simulink model "cvoo_g19_servomecanismo_atuador"  (R2022a)
settings: Solver=VariableStepAuto  StartTime=0.0  StopTime=100  RelTol=1e-3
values from neighbouring files (symbols this model uses):
  b_h_pt = [ ... (first row only)    [Ponto3.m]    (also in main.m; main_novo.m)
  c_h_pt = eye(size(a_h_pt))    [Ponto3.m]    (also in main.m; main_novo.m)
  conv_max = 5    [main.m]    (also in main_novo.m)
  conv_min = 0    [main.m]    (also in main_novo.m)
  conv_rms = 1.5*conv_res    (= 0.000915639116103)    [main.m]    (also in main_novo.m)
  d_h_pt = zeros(size(b_h_pt))    [Ponto3.m]    (also in main.m; main_novo.m)
  deg = pi/180    (= 0.0174532925199)    [Ponto3.m]    (also in def_model.m; def_model_inicial.m; main.m; main_controlo_altitude.m)
  f_amost = 100    [main.m]    (also in main_novo.m)
  G_sensq = (V_max_sensq-V_min_sensq)/(q_max_sensq-q_min_sensq)    (= 0.006)    [main.m]    (also in main_novo.m)
  Gp_din = (v_pdin_max-v_pdin_min)/(pdin_max-pdin_min)    (= 0.00125)    [main.m]    (also in main_novo.m)
  h_pt_ref = -4    [Ponto3.m]    (also in main.m = -1; main_novo.m = 0)
  K_lqr = lqr(a_h_pt_int, b_h_pt_int, Q, R)    [Ponto3.m]    (also in main.m; main_controlo_altitude.m = lqr(a_h_int, b_h_sf_int, Q, R); main_novo.m)
  offset_pdin = 2.5    [main.m]    (also in main_novo.m)
  Offset_sensq = 2.5    [main.m]    (also in main_novo.m)
  p_din_tau = 0.01    [main.m]    (also in main_novo.m)
  pdin_max = 2e3    (= 2000)    [main.m]    (also in main_novo.m)
  pdin_min = -2e3    (= -2000)    [main.m]    (also in main_novo.m)
  q_max_sensq = 300    [main.m]    (also in main_novo.m)
  q_min_sensq = -300    [main.m]    (also in main_novo.m)
  rad = 180/pi    (= 57.2957795131)    [Ponto3.m]    (also in main.m; main_controlo_altitude.m; main_novo.m)
  rho0 = 1.225    [main.m]    (also in main_novo.m)
  rms_sensq = 4.4    [main.m]    (also in main_novo.m)
  tau = 0.1    [main.m]    (also in main_novo.m)
  u_ref = 1.5    [Ponto3.m]    (also in main.m = 2; main_controlo_altitude.m = -5; main_novo.m = 0)
  vel_max_at = 60    [main.m]    (also in main_novo.m)
  x0 = [0 0 0 0]    [Ponto3.m]    (also in main.m; main_controlo_altitude.m; main_novo.m)
undefined symbols (not defined in the file or in its folder): a_h_pt, cond_ini, max_deflec
libraries: simulink x3
settings Model: Creator=josem  LastModifiedBy=franc
settings SolverCC: AlgebraicLoopSolver=TrustRegion
settings DebuggingCC: UnconnectedInputMsg=warning  UnconnectedOutputMsg=warning  UnconnectedLineMsg=warning  SFMachineParentedDataDiag=warning
settings RTWCC: DLArmComputeVersion=19.05

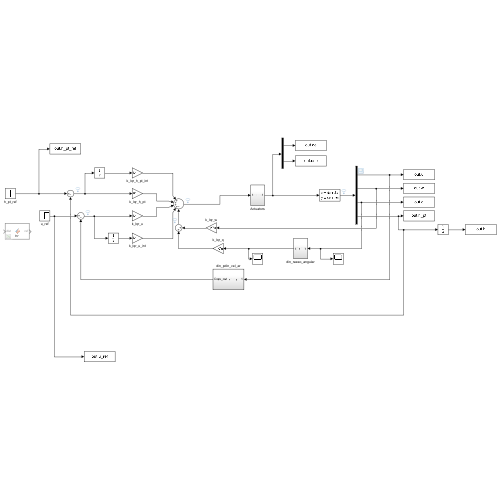
[thumbnail: Simulink's stored preview of the top-level diagram]
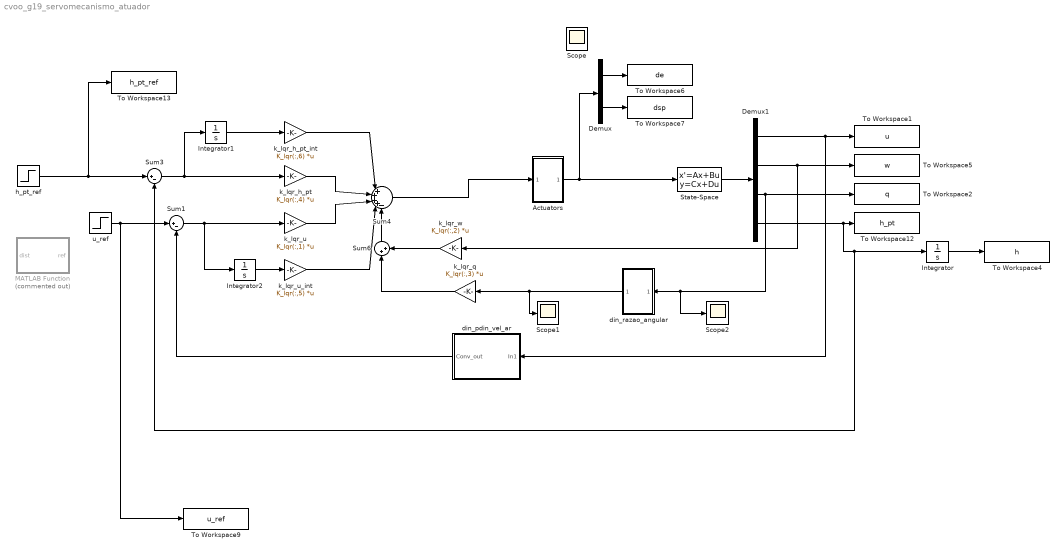
== system cvoo_g19_servomecanismo_atuador ==
  Actuators : Subsystem
  Demux : Demux  Outputs=2
  Demux1 : Demux
  Integrator : Integrator
  Integrator1 : Integrator
  Integrator2 : Integrator
  MATLAB Function : MATLAB Function  Commented=on  TreatAsAtomicUnit=on
  Scope1 : Scope
  Scope2 : Scope
  State-Space : StateSpace  A=a_h_pt  B=b_h_pt  C=c_h_pt  D=d_h_pt  InitialCondition=x0
  Sum1 : Sum  Inputs=|+-
  Sum3 : Sum  Inputs=|+-
  Sum4 : Sum  Inputs=|++++-
  Sum6 : Sum  Inputs=|++
  To Workspace1 : ToWorkspace  VariableName=u  SampleTime=-1
  To Workspace12 : ToWorkspace  VariableName=h_pt  SampleTime=-1
  To Workspace13 : ToWorkspace  VariableName=h_pt_ref  SampleTime=-1
  To Workspace2 : ToWorkspace  VariableName=q  SampleTime=-1
  To Workspace4 : ToWorkspace  VariableName=h  SampleTime=-1
  To Workspace5 : ToWorkspace  VariableName=w  SampleTime=-1
  To Workspace6 : ToWorkspace  VariableName=de  SaveFormat=Structure With Time  SampleTime=-1
  To Workspace7 : ToWorkspace  VariableName=dsp  SaveFormat=Structure With Time  SampleTime=-1
  To Workspace9 : ToWorkspace  VariableName=u_ref  SampleTime=-1
  din_pdin_vel_ar : Subsystem
  din_razao_angular : Subsystem
  h_pt_ref : Step  Time=10  After=h_pt_ref  SampleTime=0  VectorParams1D=off
  k_lqr_h_pt : Gain  Gain=K_lqr(:,4)  Multiplication=Matrix(K*u)
  k_lqr_h_pt_int : Gain  Gain=K_lqr(:,6)  Multiplication=Matrix(K*u)
  k_lqr_q : Gain  Gain=K_lqr(:,3)  Multiplication=Matrix(K*u)
  k_lqr_u : Gain  Gain=K_lqr(:,1)  Multiplication=Matrix(K*u)
  k_lqr_u_int : Gain  Gain=K_lqr(:,5)  Multiplication=Matrix(K*u)
  k_lqr_w : Gain  Gain=K_lqr(:,2)  Multiplication=Matrix(K*u)
  u_ref : Step  Time=50  After=u_ref  SampleTime=0  VectorParams1D=off
  Scope : Scope
  wires:
  State-Space/1 -> Demux1/1
  Demux1/2 -> To Workspace5/1, k_lqr_w/1
  k_lqr_h_pt/1 -> Sum4/2
  k_lqr_w/1 -> Sum6/2
  k_lqr_q/1 -> Sum6/1
  Sum6/1 -> Sum4/5
  Demux/1 -> To Workspace6/1
  Demux/2 -> To Workspace7/1
  Demux1/4 -> Integrator/1, Sum3/2, To Workspace12/1
  Integrator/1 -> To Workspace4/1
  u_ref/1 -> To Workspace9/1, Sum1/1
  Demux1/1 -> din_pdin_vel_ar/1(In1), To Workspace1/1
  k_lqr_u/1 -> Sum4/3
  Sum3/1 -> Integrator1/1, k_lqr_h_pt/1
  h_pt_ref/1 -> Sum3/1, To Workspace13/1
  Integrator1/1 -> k_lqr_h_pt_int/1
  k_lqr_h_pt_int/1 -> Sum4/1
  k_lqr_u_int/1 -> Sum4/4
  Sum1/1 -> Integrator2/1, k_lqr_u/1
  Integrator2/1 -> k_lqr_u_int/1
  Sum4/1 -> Actuators/1(In1)
  Actuators/1(Out1) -> State-Space/1, Demux/1
  Demux1/3 -> din_razao_angular/1(In1), Scope2/1, To Workspace2/1
  din_razao_angular/1(Out1) -> Scope1/1, k_lqr_q/1
  din_pdin_vel_ar/1(Conv_out) -> Sum1/2

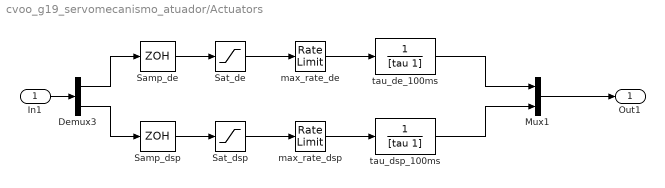
== system cvoo_g19_servomecanismo_atuador/Actuators ==
  In1 : Inport
  " max_rate_de" : RateLimiter  RisingSlewLimit=vel_max_at*deg  FallingSlewLimit=-vel_max_at*deg  SampleTimeMode=inherited
  " max_rate_dsp" : RateLimiter  RisingSlewLimit=vel_max_at*deg  FallingSlewLimit=-vel_max_at*deg  SampleTimeMode=inherited
  Demux3 : Demux  Outputs=2
  Mux1 : Mux  Inputs=2
  Samp_de : ZeroOrderHold  SampleTime=1/f_amost
  Samp_dsp : ZeroOrderHold  SampleTime=1/f_amost
  Sat_de : Saturate  UpperLimit=max_deflec.demax  LowerLimit=max_deflec.demin
  Sat_dsp : Saturate  UpperLimit=max_deflec.spmax  LowerLimit=0
  tau_de_100ms : TransferFcn  Denominator=[tau 1]
  tau_dsp_100ms : TransferFcn  Denominator=[tau 1]
  Out1 : Outport
  wires:
  Mux1/1 -> Out1/1
  In1/1 -> Demux3/1
  Sat_dsp/1 -> " max_rate_dsp"/1
  Sat_de/1 -> " max_rate_de"/1
  Demux3/1 -> Samp_de/1
  Demux3/2 -> Samp_dsp/1
  Samp_dsp/1 -> Sat_dsp/1
  Samp_de/1 -> Sat_de/1
  " max_rate_de"/1 -> tau_de_100ms/1
  " max_rate_dsp"/1 -> tau_dsp_100ms/1
  tau_dsp_100ms/1 -> Mux1/2
  tau_de_100ms/1 -> Mux1/1

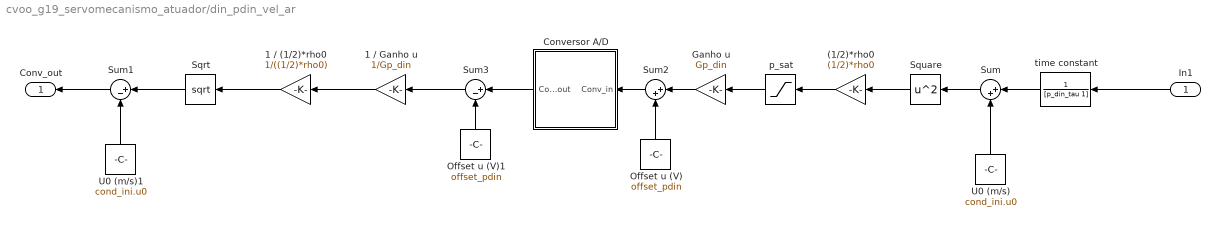
== system cvoo_g19_servomecanismo_atuador/din_pdin_vel_ar ==
  In1 : Inport
  " time constant" : TransferFcn  Denominator=[p_din_tau 1]
  (1/2)*rho0 : Gain  Gain=(1/2)*rho0
  1 / (1/2)*rho0 : Gain  Gain=1/((1/2)*rho0)
  1 / Ganho u : Gain  Gain=1/Gp_din
  Conversor A/D : Subsystem
  Ganho u : Gain  Gain=Gp_din
  Offset u (V) : Constant  Value=offset_pdin
  Offset u (V)1 : Constant  Value=offset_pdin
  Sqrt : Sqrt
  Square : Math  Operator=square  SignedPower=on
  Sum : Sum  Inputs=|++
  Sum1 : Sum  Inputs=|+-
  Sum2 : Sum  Inputs=|++
  Sum3 : Sum  Inputs=|+-
  U0 (m/s) : Constant  Value=cond_ini.u0
  U0 (m/s)1 : Constant  Value=cond_ini.u0
  p_sat : Saturate  UpperLimit=pdin_max  LowerLimit=pdin_min
  Conv_out : Outport
  wires:
  In1/1 -> " time constant"/1
  Sum/1 -> Square/1
  Ganho u/1 -> Sum2/1
  Offset u (V)/1 -> Sum2/2
  " time constant"/1 -> Sum/1
  (1/2)*rho0/1 -> p_sat/1
  U0 (m/s)/1 -> Sum/2
  p_sat/1 -> Ganho u/1
  Square/1 -> (1/2)*rho0/1
  Sum2/1 -> Conversor A/D/1(Conv_in)
  Offset u (V)1/1 -> Sum3/2
  U0 (m/s)1/1 -> Sum1/2
  Sqrt/1 -> Sum1/1
  1 / (1/2)*rho0/1 -> Sqrt/1
  1 / Ganho u/1 -> 1 / (1/2)*rho0/1
  Sum3/1 -> 1 / Ganho u/1
  Conversor A/D/1(Conv_out) -> Sum3/1
  Sum1/1 -> Conv_out/1

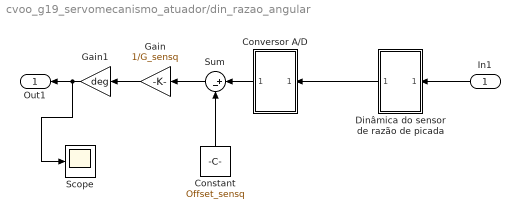
== system cvoo_g19_servomecanismo_atuador/din_razao_angular ==
  In1 : Inport
  Constant : Constant  Value=Offset_sensq
  Conversor A/D : Subsystem
  Dinâmica do sensor de razão de picada : Subsystem
  Gain : Gain  Gain=1/G_sensq
  Gain1 : Gain  Gain=deg
  Scope : Scope
  Sum : Sum  Inputs=|+-
  Out1 : Outport
  wires:
  In1/1 -> Dinâmica do sensor de razão de picada/1(In1)
  Dinâmica do sensor de razão de picada/1(Out1) -> Conversor A/D/1(In1)
  Conversor A/D/1(Out1) -> Sum/1
  Sum/1 -> Gain/1
  Constant/1 -> Sum/2
  Gain/1 -> Gain1/1
  Gain1/1 -> Scope/1, Out1/1

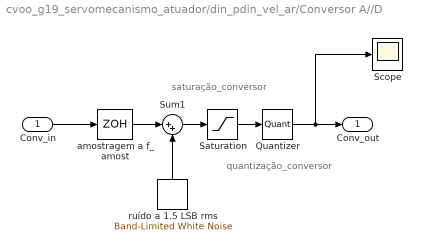
== system cvoo_g19_servomecanismo_atuador/din_pdin_vel_ar/Conversor A//D ==
  note: saturação_conversor
  note: quantização_conversor
  Conv_in : Inport
  Quantizer : Quantizer  QuantizationInterval=fat_quant
  Saturation : Saturate  UpperLimit=conv_max  LowerLimit=conv_min
  Scope : Scope
  Sum1 : Sum  Inputs=|++
  amostragem a f_amost : ZeroOrderHold  SampleTime=1/f_amost
  ruído a 1.5 LSB rms : simulink/Sources/Band-Limited White Noise  Cov=[conv_rms^2/f_amost]  Ts=1/f_amost  seed=[23341]
  Conv_out : Outport
  wires:
  Conv_in/1 -> amostragem a f_amost/1
  amostragem a f_amost/1 -> Sum1/1
  ruído a 1.5 LSB rms/1 -> Sum1/2
  Saturation/1 -> Quantizer/1
  Sum1/1 -> Saturation/1
  Quantizer/1 -> Scope/1, Conv_out/1

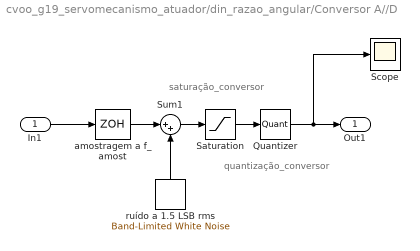
== system cvoo_g19_servomecanismo_atuador/din_razao_angular/Conversor A//D ==
  note: saturação_conversor
  note: quantização_conversor
  In1 : Inport
  Quantizer : Quantizer  QuantizationInterval=fat_quant
  Saturation : Saturate  UpperLimit=conv_max  LowerLimit=conv_min
  Scope : Scope
  Sum1 : Sum  Inputs=|++
  amostragem a f_amost : ZeroOrderHold  SampleTime=1/f_amost
  ruído a 1.5 LSB rms : simulink/Sources/Band-Limited White Noise  Cov=[conv_rms^2/f_amost]  Ts=1/f_amost  seed=[23341]
  Out1 : Outport
  wires:
  In1/1 -> amostragem a f_amost/1
  amostragem a f_amost/1 -> Sum1/1
  ruído a 1.5 LSB rms/1 -> Sum1/2
  Saturation/1 -> Quantizer/1
  Sum1/1 -> Saturation/1
  Quantizer/1 -> Scope/1, Out1/1

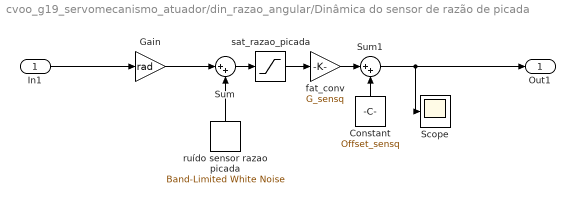
== system cvoo_g19_servomecanismo_atuador/din_razao_angular/Dinâmica do sensor de razão de picada ==
  In1 : Inport
  Constant : Constant  Value=Offset_sensq
  Gain : Gain  Gain=rad
  Scope : Scope
  Sum : Sum  Inputs=|++
  Sum1 : Sum  Inputs=|++
  fat_conv : Gain  Gain=G_sensq
  ruído sensor razao picada : simulink/Sources/Band-Limited White Noise  Cov=[rms_sensq^2/f_amost]  Ts=1/f_amost  seed=[23341]
  sat_razao_picada : Saturate  UpperLimit=q_max_sensq  LowerLimit=q_min_sensq
  Out1 : Outport
  wires:
  ruído sensor razao picada/1 -> Sum/2
  Sum1/1 -> Scope/1, Out1/1
  In1/1 -> Gain/1
  Sum/1 -> sat_razao_picada/1
  Constant/1 -> Sum1/2
  fat_conv/1 -> Sum1/1
  sat_razao_picada/1 -> fat_conv/1
  Gain/1 -> Sum/1

== matlab function cvoo_g19_servomecanismo_atuador/MATLAB Function ==
  data: dist input; ref output
function ref = fcn(dist)

dist_aux = 40*u0:10*u0:60*u0;
ref_aux = 0:2.5*u0:5*u0;
p = polyfit(dist_aux,ref_aux,2);

syms dist
ref = piecewise((dist >= 0) & (dist < 20*u0),-dist/4 + 5*u0,(dist >= 20*u0) & (dist < 40*u0),0,(dist >= 40*u0) & (dist < 60*u0),p(1)*ref^2 + p(2)*ref + p(3),(dist >= 60*u0) & (dist <= 80*u0),5*u0);

ref = piecewise((dist >= 0) & (dist < 20*u0),-dist/4 + 5*u0,(dist >= 20*u0) & (dist < 40*u0),0,(dist >= 40*u0) & (dist < 50*u0),-sqrt((2.5*u0)^2-dist^2),(dist >= 50*u0) & (dist < 60*u0),sqrt((2.5*u0)^2-dist^2),(dist >= 60*u0) & (dist <= 80*u0),5*u0);


fplot(ref)

if dist >= 0 && dist < 20*u0
    ref = -dist/4 + 5*u0;
elseif dist >= 20*u0 && dist < 40*u0
    ref = 0;
elseif dist >= 40*u0 && dist < 60*u0
    dist_aux = 40*u0:10*u0:60*u0
    ref_aux = 0:2.5*u0:5*u0
    p = polyfit(x,y,3);
    ref = p(1)*ref^3 + p(2)*ref^2 + p(3)*ref + p(4)
elseif dist >= 60*u0 && dist <= 80*u0
    ref = 5*u0
end
